simulink model "SAME5xPIM_MCLV2_MotorControl_ExtMode"  (R2021a)
settings: Solver=FixedStepDiscrete  StartTime=0.0  StopTime=inf  FixedStep=5e-5  RelTol=1e-3  EnableMultiTasking=on
InitFcn:
  | % DC Voltage
  | VDC = 24;
  | 
  | % Intersective PMW
  | Vmax = VDC/2;
  | Imax = 4;
  | 
  | Ts = 1e-4;
  | 
  | 
  | % pole paires
  | p = 4;
  | 
  | % QEI
  | lines = 4*1000;
  | eleclines = lines/p;
  | inveleclines = 1/eleclines
  | gainQEIspeed = 2*pi/Ts/lines
  | 
  | % Electrical parameters
  | R=0.656; L=0.35e-3; Phif=0.0066;
  | % Mechanical parameters
  | F=1.e-05; J=1e-05; C0 = 0.01;%10;%1;
undefined symbols (not defined in the file or in its folder): ADC0, AIN0, AIN6, B27, DiscIntNeverNeededParam, PA02, PA03, PA06, PA08, PA09, PA10, PA11, PA12, PA13, PA16, PA17, PA18, pad0, pad1, pad2, pad3, PB08, PC16, PC17, PC18, Pin, SAME54P20A, TQFP128, VREFA, wo0, wo1, wo2, wo4, wo5, wo6
libraries: simulink x15, MCHP_Blockset x9, dsparch4 x1
(part 2 of 2)

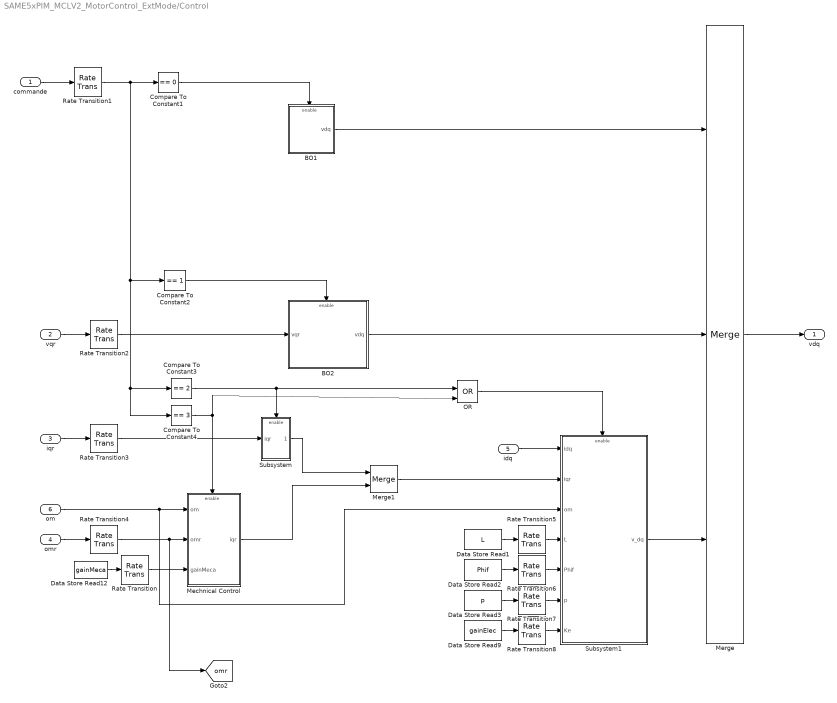
== system SAME5xPIM_MCLV2_MotorControl_ExtMode/Control ==
  commande : Inport
  vqr : Inport  Port=2
  iqr : Inport  Port=3
  omr : Inport  Port=4
  idq : Inport  Port=5
  om : Inport  Port=6
  BO1 : Subsystem
  BO2 : Subsystem
  Compare To Constant1 : simulink/Logic and Bit Operations/Compare To Constant  relop===  const=0  OutDataTypeStr=boolean
  Compare To Constant2 : simulink/Logic and Bit Operations/Compare To Constant  relop===  const=1  OutDataTypeStr=boolean
  Compare To Constant3 : simulink/Logic and Bit Operations/Compare To Constant  relop===  const=2  OutDataTypeStr=boolean
  Compare To Constant4 : simulink/Logic and Bit Operations/Compare To Constant  relop===  const=3  OutDataTypeStr=boolean
  Data Store Read1 : DataStoreRead  DataStoreName=L  SampleTime=1  IndexOptions=Index vector (dialog)  Indices=1  OutputSizes=1
  Data Store Read12 : DataStoreRead  DataStoreName=gainMeca  SampleTime=1  IndexOptions=Index vector (dialog)  Indices=1  OutputSizes=1
  Data Store Read2 : DataStoreRead  DataStoreName=Phif  SampleTime=1  IndexOptions=Index vector (dialog)  Indices=1  OutputSizes=1
  Data Store Read3 : DataStoreRead  DataStoreName=p  SampleTime=1  IndexOptions=Index vector (dialog)  Indices=1  OutputSizes=1
  Data Store Read9 : DataStoreRead  DataStoreName=gainElec  SampleTime=1  IndexOptions=Index vector (dialog)  Indices=1  OutputSizes=1
  Mechnical Control : Subsystem
  Merge : Merge  Inputs=3
  Merge1 : Merge
  OR : Logic  Operator=OR  IconShape=distinctive  AllPortsSameDT=off  OutDataTypeStr=boolean
  Rate Transition{,1..8} (9 alike) : RateTransition
  Subsystem : Subsystem
  Subsystem1 : Subsystem
  vdq : Outport  VectorParamsAs1DForOutWhenUnconnected=off
  tag scope: omr=global
  wires:
  Data Store Read12/1 -> Rate Transition/1
  omr/1 -> Rate Transition4/1
  iqr/1 -> Rate Transition3/1
  vqr/1 -> Rate Transition2/1
  Data Store Read2/1 -> Rate Transition6/1
  Data Store Read3/1 -> Rate Transition7/1
  Data Store Read1/1 -> Rate Transition5/1
  Data Store Read9/1 -> Rate Transition8/1
  BO2/1(vdq) -> Merge/2
  BO1/1(vdq) -> Merge/1
  Compare To Constant2/1 -> BO2/Enable
  Merge/1 -> vdq/1
  commande/1 -> Rate Transition1/1
  Compare To Constant1/1 -> BO1/Enable
  Compare To Constant3/1 -> OR/1, Subsystem/Enable
  Rate Transition1/1 -> Compare To Constant2/1, Compare To Constant3/1, Compare To Constant4/1, Compare To Constant1/1
  Subsystem/1(Out1) -> Merge1/1
  Mechnical Control/1(iqr) -> Merge1/2
  Compare To Constant4/1 -> OR/2, Mechnical Control/Enable
  om/1 -> Subsystem1/3(om), Mechnical Control/1(om)
  OR/1 -> Subsystem1/Enable
  idq/1 -> Subsystem1/1(idq)
  Merge1/1 -> Subsystem1/2(iqr)
  Subsystem1/1(v_dq) -> Merge/3
  Rate Transition2/1 -> BO2/1(vqr)
  Rate Transition3/1 -> Subsystem/1(iqr)
  Rate Transition4/1 -> Mechnical Control/2(omr), [omr]
  Rate Transition/1 -> Mechnical Control/3(gainMeca)
  Rate Transition5/1 -> Subsystem1/4(L)
  Rate Transition6/1 -> Subsystem1/5(Phif)
  Rate Transition7/1 -> Subsystem1/6(p)
  Rate Transition8/1 -> Subsystem1/7(Ke)

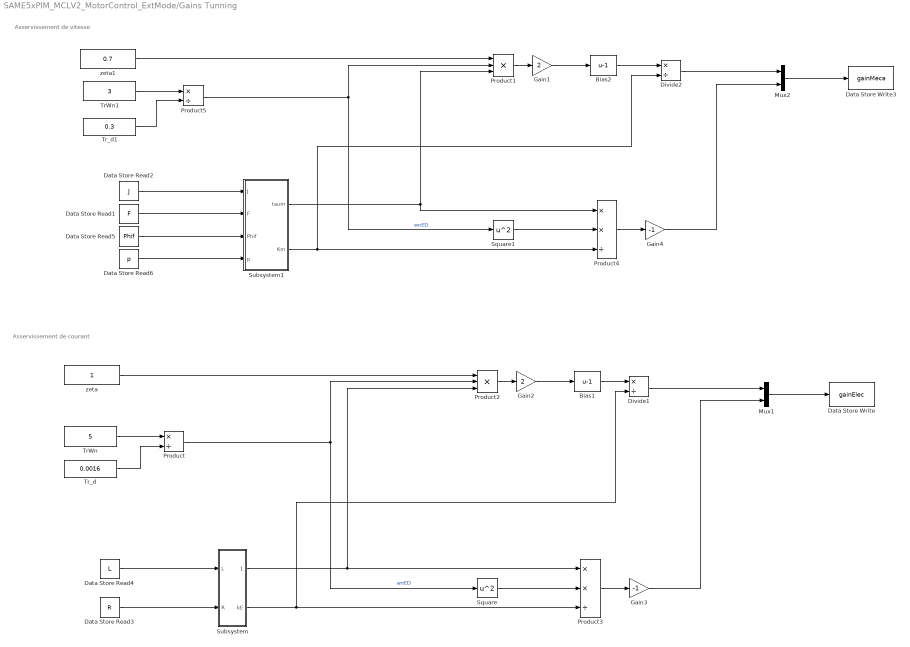
== system SAME5xPIM_MCLV2_MotorControl_ExtMode/Gains Tunning ==
  note: Asservissement de vitesse
  note: Asservissement de courant
  Bias1 : Bias  Bias=-1
  Bias2 : Bias  Bias=-1
  Data Store Read1 : DataStoreRead  DataStoreName=F  SampleTime=1  IndexOptions=Index vector (dialog)  Indices=1  OutputSizes=1
  Data Store Read2 : DataStoreRead  DataStoreName=J  SampleTime=1  IndexOptions=Index vector (dialog)  Indices=1  OutputSizes=1
  Data Store Read3 : DataStoreRead  DataStoreName=R  SampleTime=1  IndexOptions=Index vector (dialog)  Indices=1  OutputSizes=1
  Data Store Read4 : DataStoreRead  DataStoreName=L  SampleTime=1  IndexOptions=Index vector (dialog)  Indices=1  OutputSizes=1
  Data Store Read5 : DataStoreRead  DataStoreName=Phif  SampleTime=1  IndexOptions=Index vector (dialog)  Indices=1  OutputSizes=1
  Data Store Read6 : DataStoreRead  DataStoreName=p  SampleTime=1  IndexOptions=Index vector (dialog)  Indices=1  OutputSizes=1
  Data Store Write : DataStoreWrite  DataStoreName=gainElec  SampleTime=1  IndexOptions=Index vector (dialog)  Indices=1  OutputSizes=1
  Data Store Write3 : DataStoreWrite  DataStoreName=gainMeca  IndexOptions=Index vector (dialog)  Indices=1  OutputSizes=1
  Divide1 : Product  Inputs=*/
  Divide2 : Product  Inputs=*/
  Gain1 : Gain  Gain=2
  Gain2 : Gain  Gain=2
  Gain3 : Gain  Gain=-1
  Gain4 : Gain  Gain=-1
  Mux1 : Mux  Inputs=2
  Mux2 : Mux  Inputs=2
  Product : Product  Inputs=*/
  Product1 : Product  Inputs=3
  Product2 : Product  Inputs=3
  Product3 : Product  Inputs=**/
  Product4 : Product  Inputs=**/
  Product5 : Product  Inputs=*/
  Square : Math  Operator=square  SaturateOnIntegerOverflow=on
  Square1 : Math  Operator=square  SaturateOnIntegerOverflow=on
  Subsystem : Subsystem
  Subsystem1 : Subsystem
  TrWn : Constant  Value=5  OutDataTypeStr=single
  TrWn1 : Constant  Value=3  OutDataTypeStr=single
  Tr_d : Constant  Value=0.0016  OutDataTypeStr=single
  Tr_d1 : Constant  Value=0.3  OutDataTypeStr=single
  zeta : Constant  OutDataTypeStr=single
  zeta1 : Constant  Value=0.7  OutDataTypeStr=single
  wires:
  Subsystem1/2(Km) -> Product4/3, Divide2/2
  Subsystem1/1(taum) -> Product1/3, Product4/1
  Product5/1 -> Product1/2, Square1/1  "wnED"
  zeta1/1 -> Product1/1
  TrWn1/1 -> Product5/1
  Tr_d1/1 -> Product5/2
  Data Store Read6/1 -> Subsystem1/4(p)
  Data Store Read5/1 -> Subsystem1/3(Phif)
  Data Store Read1/1 -> Subsystem1/2(F)
  Data Store Read2/1 -> Subsystem1/1(J)
  Mux2/1 -> Data Store Write3/1
  Gain4/1 -> Mux2/2
  Product4/1 -> Gain4/1
  Divide2/1 -> Mux2/1
  Bias2/1 -> Divide2/1
  Product1/1 -> Gain1/1
  Gain1/1 -> Bias2/1
  Square1/1 -> Product4/2
  Square/1 -> Product3/2
  zeta/1 -> Product2/1
  Gain2/1 -> Bias1/1
  Subsystem/2(kE) -> Product3/3, Divide1/2
  Product/1 -> Square/1, Product2/2  "wnED"
  Tr_d/1 -> Product/2
  TrWn/1 -> Product/1
  Subsystem/1(tauE) -> Product3/1, Product2/3
  Data Store Read3/1 -> Subsystem/2(R)
  Data Store Read4/1 -> Subsystem/1(L)
  Mux1/1 -> Data Store Write/1
  Product2/1 -> Gain2/1
  Bias1/1 -> Divide1/1
  Divide1/1 -> Mux1/1
  Product3/1 -> Gain3/1
  Gain3/1 -> Mux1/2

== system SAME5xPIM_MCLV2_MotorControl_ExtMode/Inv Park ==
  cossin : Inport
  vdq : Inport  Port=2  PortDimensions=2
  Clakeinv : Subsystem
  ParkInv : Subsystem
  vabc : Outport  VectorParamsAs1DForOutWhenUnconnected=off
  wires:
  Clakeinv/1(abc) -> vabc/1
  ParkInv/1(valbe) -> Clakeinv/1(alphabeta)
  cossin/1 -> ParkInv/1(cos(pth)sin(pth))
  vdq/1 -> ParkInv/2(vdq)

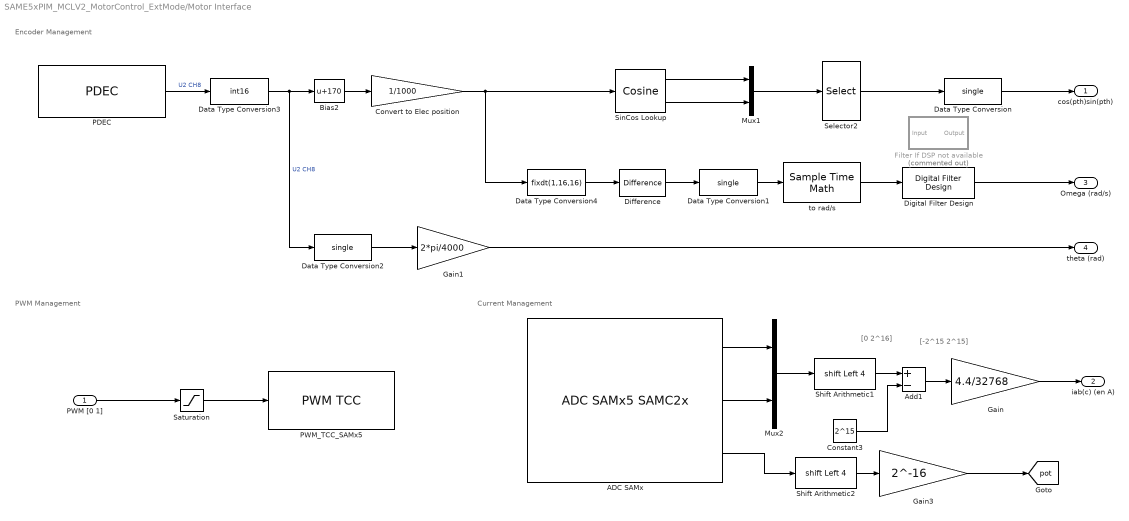
== system SAME5xPIM_MCLV2_MotorControl_ExtMode/Motor Interface ==
  note: Current Management
  note: [-2^15 2^15]
  note: [0 2^16]
  note: PWM Management
  note: Encoder Management
  PWM [0 1] : Inport
  ADC SAMx : MCHP_Blockset/Analog IO/ADC SAMx5 SAMC2x  ADCREF=ADC 0 and ADC 1 (slave)  VREF_seq0=Dynamic Options  VREF_seq0_TXT=PA03 / VREFA / Pin[10]  info=0  SampleTime=1e-4  MCHP_PORT={ADC0_seq0.0}{ADC0_AIN0}15:2:P2;{ADC0_seq1.0}{ADC0_AIN6}15:2:P6;{ADC1_seq0.0}{ADC1_AIN0}15:2:P40;  MCHP_MASTERLINK=SAME5xPIM_MCLV2_MotorControl_ExtMode/Microchip Master  MCHP_CRC=4644056  TrigSource_seq0=Dynamic Options  TrigSource_seq0_TXT=TCC0 PWM event Overflow - Period  ADC0_seq0=Dynamic Options  ADC0_seq0_TXT=PA02 / AIN0 / Pin[9]  ADC1_seq0=Dynamic Options  ADC1_seq0_TXT=PB08 / AIN0 / Pin[19]  ADC0_seq0_1=Dynamic Options  ADC0_seq0_1_TXT=Not Used  ADC1_seq0_1=Dynamic Options  ADC1_seq0_1_TXT=Not Used  ADC0_seq0_2=Dynamic Options  ADC0_seq0_2_TXT=Not Used  ADC1_seq0_2=Dynamic Options  ADC1_seq0_2_TXT=Not Used  ADC0_seq0_3=Dynamic Options  ADC0_seq0_3_TXT=Not Used  ADC1_seq0_3=Dynamic Options  ADC1_seq0_3_TXT=Not Used  ADC0_seq0_4=Dynamic Options  ADC0_seq0_4_TXT=Not Used  ADC1_seq0_4=Dynamic Options  ADC1_seq0_4_TXT=Not Used  ADC0_seq0_5=Dynamic Options  ADC0_seq0_5_TXT=Not Used  ADC1_seq0_5=Dynamic Options  ADC1_seq0_5_TXT=Not Used  Resolution_seq0=12 bits  SampleTime_seq0_s=1e-6  TrigTimeStep_seq0=on  info_seq0=0  TrigSource_seq1=Dynamic Options  TrigSource_seq1_TXT=after previous sequence  ADC0_seq1=Dynamic Options  ADC0_seq1_TXT=PA06 / AIN6 / Pin[23]  ADC1_seq1=Dynamic Options  ADC1_seq1_TXT=Not Used  ADC0_seq1_1=Dynamic Options  ADC0_seq1_1_TXT=Not Used  ADC1_seq1_1=Dynamic Options  ADC1_seq1_1_TXT=Not Used  ADC0_seq1_2=Dynamic Options  ADC0_seq1_2_TXT=Not Used  ADC1_seq1_2=Dynamic Options  ADC1_seq1_2_TXT=Not Used  ADC0_seq1_3=Dynamic Options  ADC0_seq1_3_TXT=Not Used  ADC1_seq1_3=Dynamic Options  ADC1_seq1_3_TXT=Not Used  ADC0_seq1_4=Dynamic Options  ADC0_seq1_4_TXT=Not Used  ADC1_seq1_4=Dynamic Options  ADC1_seq1_4_TXT=Not Used  ADC0_seq1_5=Dynamic Options  ADC0_seq1_5_TXT=Not Used  ADC1_seq1_5=Dynamic Options  ADC1_seq1_5_TXT=Not Used  Resolution_seq1=12 bits  SampleTime_seq1_s=1e-6  TrigTimeStep_seq1=off  info_seq1=0  TrigSource_seq2=Dynamic Options  TrigSource_seq2_TXT=after previous sequence  ADC0_seq2=Dynamic Options  ADC0_seq2_TXT=Not Used  ADC1_seq2=Dynamic Options  ADC1_seq2_TXT=Not Used  ADC0_seq2_1=Dynamic Options  ADC0_seq2_1_TXT=Not Used  ADC1_seq2_1=Dynamic Options  ADC1_seq2_1_TXT=Not Used  ADC0_seq2_2=Dynamic Options  ADC0_seq2_2_TXT=Not Used  ADC1_seq2_2=Dynamic Options  ADC1_seq2_2_TXT=Not Used  ADC0_seq2_3=Dynamic Options  ADC0_seq2_3_TXT=Not Used  ADC1_seq2_3=Dynamic Options  ADC1_seq2_3_TXT=Not Used  ADC0_seq2_4=Dynamic Options  ADC0_seq2_4_TXT=Not Used  ADC1_seq2_4=Dynamic Options  ADC1_seq2_4_TXT=Not Used  ADC0_seq2_5=Dynamic Options  ADC0_seq2_5_TXT=Not Used  ADC1_seq2_5=Dynamic Options  ADC1_seq2_5_TXT=Not Used  Resolution_seq2=12 bits  SampleTime_seq2_s=1e-6  TrigTimeStep_seq2=off  info_seq2=0  TrigSource_seq3=Dynamic Options  TrigSource_seq3_TXT=after previous sequence  ADC0_seq3=Dynamic Options  ADC0_seq3_TXT=Not Used  ADC1_seq3=Dynamic Options  ADC1_seq3_TXT=Not Used  ADC0_seq3_1=Dynamic Options  ADC0_seq3_1_TXT=Not Used  ADC1_seq3_1=Dynamic Options  ADC1_seq3_1_TXT=Not Used  ADC0_seq3_2=Dynamic Options  ADC0_seq3_2_TXT=Not Used  ADC1_seq3_2=Dynamic Options  ADC1_seq3_2_TXT=Not Used  ADC0_seq3_3=Dynamic Options  ADC0_seq3_3_TXT=Not Used  ADC1_seq3_3=Dynamic Options  ADC1_seq3_3_TXT=Not Used  ADC0_seq3_4=Dynamic Options  ADC0_seq3_4_TXT=Not Used  ADC1_seq3_4=Dynamic Options  ADC1_seq3_4_TXT=Not Used  ADC0_seq3_5=Dynamic Options  ADC0_seq3_5_TXT=Not Used  ADC1_seq3_5=Dynamic Options  ADC1_seq3_5_TXT=Not Used  Resolution_seq3=12 bits  SampleTime_seq3_s=1e-6  TrigTimeStep_seq3=off  info_seq3=0  TrigSource_seq4=Dynamic Options  TrigSource_seq4_TXT=after previous sequence  ADC0_seq4=Dynamic Options  ADC0_seq4_TXT=Not Used  ADC1_seq4=Dynamic Options  ADC1_seq4_TXT=Not Used  ADC0_seq4_1=Dynamic Options  ADC0_seq4_1_TXT=Not Used  ADC1_seq4_1=Dynamic Options  ADC1_seq4_1_TXT=Not Used  ADC0_seq4_2=Dynamic Options  ADC0_seq4_2_TXT=Not Used  ADC1_seq4_2=Dynamic Options  ADC1_seq4_2_TXT=Not Used  ADC0_seq4_3=Dynamic Options  ADC0_seq4_3_TXT=Not Used  ADC1_seq4_3=Dynamic Options  ADC1_seq4_3_TXT=Not Used  ADC0_seq4_4=Dynamic Options  ADC0_seq4_4_TXT=Not Used  ADC1_seq4_4=Dynamic Options  ADC1_seq4_4_TXT=Not Used  ADC0_seq4_5=Dynamic Options  ADC0_seq4_5_TXT=Not Used  ADC1_seq4_5=Dynamic Options  ADC1_seq4_5_TXT=Not Used  Resolution_seq4=12 bits  SampleTime_seq4_s=1e-6  TrigTimeStep_seq4=off  info_seq4=0  TrigSource_seq5=Dynamic Options  TrigSource_seq5_TXT=after previous sequence  ADC0_seq5=Dynamic Options  ADC0_seq5_TXT=Not Used  ADC1_seq5=Dynamic Options  ADC1_seq5_TXT=Not Used  ADC0_seq5_1=Dynamic Options  ADC0_seq5_1_TXT=Not Used  ADC1_seq5_1=Dynamic Options  ADC1_seq5_1_TXT=Not Used  ADC0_seq5_2=Dynamic Options  ADC0_seq5_2_TXT=Not Used  ADC1_seq5_2=Dynamic Options  ADC1_seq5_2_TXT=Not Used  ADC0_seq5_3=Dynamic Options  ADC0_seq5_3_TXT=Not Used  ADC1_seq5_3=Dynamic Options  ADC1_seq5_3_TXT=Not Used  ADC0_seq5_4=Dynamic Options  ADC0_seq5_4_TXT=Not Used  ADC1_seq5_4=Dynamic Options  ADC1_seq5_4_TXT=Not Used  ADC0_seq5_5=Dynamic Options  ADC0_seq5_5_TXT=Not Used  ADC1_seq5_5=Dynamic Options  ADC1_seq5_5_TXT=Not Used  Resolution_seq5=12 bits  SampleTime_seq5_s=1e-6  TrigTimeStep_seq5=off  info_seq5=0
      settings: SourceProductName=MPLAB Device Blocks for Simulink
  Add1 : Sum  Inputs=+-  OutDataTypeStr=single
  Bias2 : Bias  Bias=170
  Constant3 : Constant  Value=2^15  OutDataTypeStr=fixdt(0,16,0)
  Convert to Elec position : Gain  Gain=1/1000  OutDataTypeStr=fixdt(0,16,16)
  Data Type Conversion : DataTypeConversion  OutDataTypeStr=single
  Data Type Conversion1 : DataTypeConversion  OutDataTypeStr=single
  Data Type Conversion2 : DataTypeConversion  OutDataTypeStr=single
  Data Type Conversion3 : DataTypeConversion  OutDataTypeStr=int16  ConvertRealWorld=Stored Integer (SI)
  Data Type Conversion4 : DataTypeConversion  OutDataTypeStr=fixdt(1,16,16)  ConvertRealWorld=Stored Integer (SI)
  Difference : simulink/Discrete/Difference  ICPrevInput=0  OutMin=[]  OutMax=[]  OutDataType=fixdt(1, 16)  OutScaling=2^-10  DoSatur=off
  Digital Filter Design : dsparch4/Digital Filter Design  mwdsp_browser_bugfix_var=off
  Filter If DSP not available : Subsystem  Tag=FilterWizardSubSystem  Commented=on
      settings: ErrorFcn=dspFilterRealizedInBasicElemsAlgLoopErrFcnCallback
  Gain : Gain  Gain=4.4/32768
  Gain1 : Gain  Gain=2*pi/4000
  Gain3 : Gain  Gain=2^-16  OutDataTypeStr=single
  Mux1 : Mux  Inputs=2
  Mux2 : Mux  Inputs=2
  PDEC : MCHP_Blockset/QEI/PDEC  Mode=Quadrature Encoder  index=Reset counter  QDI0=PC16 / Pin[70]  QDI0_txt=Dynamic Options  QDI1=PC17 / Pin[71]  QDI1_txt=Dynamic Options  QDI2=PC18 / Pin[72]  QDI2_txt=Dynamic Options  maxCounterReset=-1  AutoCorrection=off  AutoCorrection_override=on  info=0  MCHP_MASTERLINK=SAME5xPIM_MCLV2_MotorControl_ExtMode/Microchip Master  SampleTime=1e-4  MCHP_PORT={PDEC A}{PDEC_QDI0}5:0:P80;{PDEC B}{PDEC_QDI1}5:0:P81;{PDEC index}{PDEC_QDI2}5:0:P82;  MAXPOS_INPUT=off  RESET_INPUT=off  OutputCounter=on  OutputCounter_Signed=unsigned  OutputRevolution=off  CounterRevolution_length=Counter is 13 bits ; revolution is 3 bits  OutputRevolution_Signed=unsigned  FILTER="250 (ns)  ->  freq 2 (MHz)"  FILTER_TXT="250 (ns)  ->  freq 2 (MHz)"  SWAP=off  QDI_invert_0=off  QDI_invert_1=off  QDI_invert_2=off
      settings: SourceProductName=MPLAB Device Blocks for Simulink
  PWM_TCC_SAMx5 : MCHP_Blockset/PWM IO/PWM TCC  TCCREF=TCC 0  WAVE_choice=Center aligned PWM  MaxPeriod_s=5e-5  OTMX=Default  WO0=Dynamic Options  WO0_TXT=PA08 / Pin[33] / wo0  WO1=Dynamic Options  WO1_TXT=PA09 / Pin[34] / wo1  WO2=Dynamic Options  WO2_TXT=PA10 / Pin[35] / wo2  WO3=Dynamic Options  WO3_TXT=Not Used  WO4=Dynamic Options  WO4_TXT=PA16 / Pin[66] / wo4  WO5=Dynamic Options  WO5_TXT=PA17 / Pin[67] / wo5  WO6=Dynamic Options  WO6_TXT=PA18 / Pin[68] / wo6  WO7=Dynamic Options  WO7_TXT=Not Used  info=0  evalin_ws=PWM0max=MCHP_Fun.Hex2num('40A76E0000000000');PWM0max=MCHP_Fun.Hex2num('40A76E0000000000');PWM0max=MCHP_Fun.Hex2num('40A76E0000000000');  SampleTime=1e-4  MCHP_PORT={PWM0_H0}{TCC0_WO0}5:1:P8;{PWM0_H1}{TCC0_WO1}5:1:P9;{PWM0_H2}{TCC0_WO2}5:1:P10;{PWM0_L0}{TCC0_WO4}5:1:P16;{PWM0_L1}{TCC0_WO5}5:1:P17;{PWM0_L2}{TCC0_WO6}5:1:P18;  MCHP_MASTERLINK=SAME5xPIM_MCLV2_MotorControl_ExtMode/Microchip Master  INVEN_WO0=off  INVEN_WO1=off  INVEN_WO2=off  INVEN_WO3=off  INVEN_WO4=off  INVEN_WO5=off  INVEN_WO6=off  INVEN_WO7=off  SWAP_PWM0=off  SWAP_PWM1=off  SWAP_PWM2=off  SWAP_PWM3=off  POL_PWM0=off  POL_PWM1=off  POL_PWM2=off  POL_PWM3=off  POL_PWM4=off  POL_PWM5=off  InitPeriod_s=5e-5  InitDutyCycle_s=2.5e-5  InitDeadTimeH_s=0.5e-6  InitDeadTimeL_s=0.5e-6  InitOutputOverride=0  InitOutputOverride_val=0  BlockInput_VectorScalar=Vectors (grouped by function)  BlockInput_Period=Not a block input  BlockInput_DutyCycle=a Floating Point input within range [0 1]  BlockInput_DeadTime=Not a block input  BlockInput_OutputOverride=Not a block input
      settings: SourceProductName=MPLAB Device Blocks for Simulink
  Saturation : Saturate  UpperLimit=0.98  LowerLimit=0.02  LinearizeAsGain=off  OutDataTypeStr=double
  Selector2 : Selector  InputPortWidth=2  IndexOptions=Index vector (dialog)  Indices=[2 1]  OutputSizes=1
  Shift Arithmetic1 : ArithShift  BitShiftNumber=4  BitShiftDirection=Left
  Shift Arithmetic2 : ArithShift  BitShiftNumber=4  BitShiftDirection=Left
  SinCos Lookup : simulink/Lookup Tables/Cosine  Formula=sin(2*pi*u) and cos(2*pi*u)  NumDataPoints=(2^12)+1  OutputWordLength=16  InternalRulePriority=Precision
      settings: SourceProductBaseCode=SL
  to rad/s : SampleTimeMath  TsampMathOp=/  weightValue=(4)/(2*pi)
  cos(pth)sin(pth) : Outport  VectorParamsAs1DForOutWhenUnconnected=off
  iab(c) (en A) : Outport  Port=2  VectorParamsAs1DForOutWhenUnconnected=off
  Omega (rad/s) : Outport  Port=3  PortDimensions=1  VectorParamsAs1DForOutWhenUnconnected=off
  theta (rad) : Outport  Port=4  VectorParamsAs1DForOutWhenUnconnected=off
  tag scope: pot=global
  wires:
  ADC SAMx/3 -> Shift Arithmetic2/1
  ADC SAMx/1 -> Mux2/1
  Constant3/1 -> Add1/2
  ADC SAMx/2 -> Mux2/2
  Shift Arithmetic1/1 -> Add1/1
  Mux2/1 -> Shift Arithmetic1/1
  Add1/1 -> Gain/1
  Gain3/1 -> [pot]
  Gain/1 -> iab(c) (en A)/1
  Shift Arithmetic2/1 -> Gain3/1
  Data Type Conversion1/1 -> to rad/s/1
  Data Type Conversion4/1 -> Difference/1
  Difference/1 -> Data Type Conversion1/1
  Gain1/1 -> theta (rad)/1
  Data Type Conversion2/1 -> Gain1/1
  Data Type Conversion3/1 -> Bias2/1, Data Type Conversion2/1  "U2 CH8"
  SinCos Lookup/1 -> Mux1/1
  SinCos Lookup/2 -> Mux1/2
  Selector2/1 -> Data Type Conversion/1
  Mux1/1 -> Selector2/1
  Data Type Conversion/1 -> cos(pth)sin(pth)/1
  Digital Filter Design/1 -> Omega (rad/s)/1
  PDEC/1 -> Data Type Conversion3/1  "U2 CH8"
  Bias2/1 -> Convert to Elec position/1
  to rad/s/1 -> Digital Filter Design/1
  Convert to Elec position/1 -> SinCos Lookup/1, Data Type Conversion4/1
  PWM [0 1]/1 -> Saturation/1
  Saturation/1 -> PWM_TCC_SAMx5/1

== system SAME5xPIM_MCLV2_MotorControl_ExtMode/PWM ==
  vabc : Inport
  50% average duty-cycle : Bias  Bias=0.5
  Gain : Gain  Gain=1/VDC  OutDataTypeStr=double
  PWM [0 1] : Outport  VectorParamsAs1DForOutWhenUnconnected=off
  wires:
  Gain/1 -> 50% average duty-cycle/1
  50% average duty-cycle/1 -> PWM [0 1]/1
  vabc/1 -> Gain/1

== system SAME5xPIM_MCLV2_MotorControl_ExtMode/Park  ==
  cossin : Inport
  xab(c) : Inport  Port=2
  Clark Fixe : Subsystem
  Park Fixe : Subsystem
  xdq : Outport  VectorParamsAs1DForOutWhenUnconnected=off
  wires:
  Park Fixe/1(xdq) -> xdq/1
  cossin/1 -> Park Fixe/2(cos(pth)sin(pth))
  xab(c)/1 -> Clark Fixe/1(xab(c))
  Clark Fixe/1(xalphabeta) -> Park Fixe/1(xalphabeta)

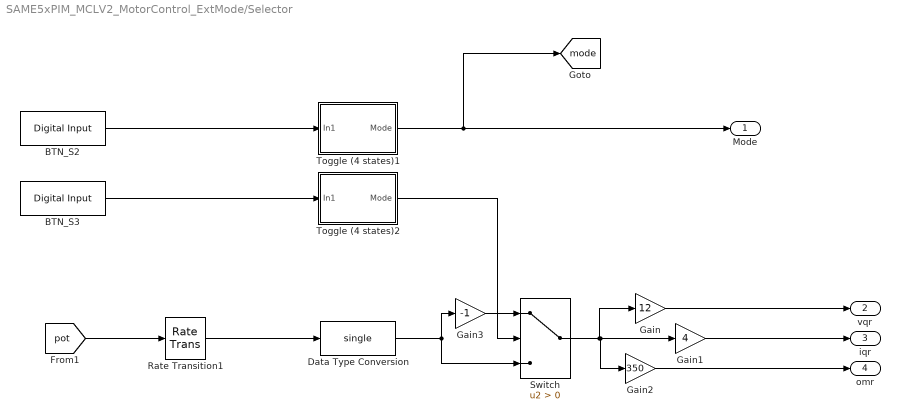
== system SAME5xPIM_MCLV2_MotorControl_ExtMode/Selector ==
  BTN_S2 : MCHP_Blockset/Digital IO/Digital Input  PORT=Dynamic Options  PORT_TXT="D   [ 0  1  8  9  10  11  12  20  21 ]"  PIN=9  PACK=off  SIMULTANEOUS=off  ORDERING=None  SampleTime=.1  MCHP_PORT={Digital In}{DIN}2:0:D9;  MCHP_MASTERLINK=SAME5xPIM_MCLV2_MotorControl_ExtMode/Microchip Master
      settings: SourceProductName=MPLAB Device Blocks for Simulink
  BTN_S3 : MCHP_Blockset/Digital IO/Digital Input  PORT=Dynamic Options  PORT_TXT="D   [ 0  1  8  9  10  11  12  20  21 ]"  PIN=10  PACK=off  SIMULTANEOUS=off  ORDERING=None  SampleTime=.1  MCHP_PORT={Digital In}{DIN}2:0:D10;  MCHP_MASTERLINK=SAME5xPIM_MCLV2_MotorControl_ExtMode/Microchip Master
      settings: SourceProductName=MPLAB Device Blocks for Simulink
  Data Type Conversion : DataTypeConversion  OutDataTypeStr=single
  Gain : Gain  Gain=12
  Gain1 : Gain  Gain=4
  Gain2 : Gain  Gain=350
  Gain3 : Gain  Gain=-1
  Rate Transition1 : RateTransition  OutPortSampleTime=0.1
  Switch : Switch  Criteria=u2 > Threshold
  Toggle (4 states)1 : Subsystem
  Toggle (4 states)2 : Subsystem
  Mode : Outport  VectorParamsAs1DForOutWhenUnconnected=off
  vqr : Outport  Port=2  VectorParamsAs1DForOutWhenUnconnected=off
  iqr : Outport  Port=3  VectorParamsAs1DForOutWhenUnconnected=off
  omr : Outport  Port=4  VectorParamsAs1DForOutWhenUnconnected=off
  tag scope: mode=global
  wires:
  Gain3/1 -> Switch/1
  Data Type Conversion/1 -> Switch/3, Gain3/1
  Toggle (4 states)2/1(Mode) -> Switch/2
  BTN_S3/1 -> Toggle (4 states)2/1(In1)
  Rate Transition1/1 -> Data Type Conversion/1
  [pot] -> Rate Transition1/1
  Toggle (4 states)1/1(Mode) -> Mode/1, [mode]
  Switch/1 -> Gain2/1, Gain1/1, Gain/1
  Gain/1 -> vqr/1
  Gain1/1 -> iqr/1
  Gain2/1 -> omr/1
  BTN_S2/1 -> Toggle (4 states)1/1(In1)

== system SAME5xPIM_MCLV2_MotorControl_ExtMode/Control/BO1 ==
  Enable : EnablePort
  Mux : Mux  Inputs=2
  vd : Constant  Value=0  OutMin=[-12]  OutMax=[12]  OutDataTypeStr=single
  vq : Constant  Value=0  OutMin=[-12]  OutMax=[12]  OutDataTypeStr=single
  vdq : Outport  VectorParamsAs1DForOutWhenUnconnected=off
  wires:
  vq/1 -> Mux/2
  Mux/1 -> vdq/1
  vd/1 -> Mux/1

== system SAME5xPIM_MCLV2_MotorControl_ExtMode/Control/BO2 ==
  vqr : Inport
  Enable : EnablePort
  Constant : Constant  Value=0  OutDataTypeStr=single
  Mux : Mux  Inputs=2
  vdq : Outport  VectorParamsAs1DForOutWhenUnconnected=off
  wires:
  Mux/1 -> vdq/1
  Constant/1 -> Mux/1
  vqr/1 -> Mux/2

== system SAME5xPIM_MCLV2_MotorControl_ExtMode/Control/Mechnical Control ==
  om : Inport
  omr : Inport  Port=2
  gainMeca : Inport  Port=3
  Enable : EnablePort  StatesWhenEnabling=reset
  Augmented state feedback : Subsystem
      settings: PortSchema="{\"entries\":[{\"content\":{\"sides\":[{\"content\":{\"connectorIds\":[\"In1\",\"In2\"]},\"type\":\"ConnectorPlacement.EquallySpacedRectSide\",\"uuid\":\"89137e2f-cd18-4dcc-a524-9caf5367be1f\"},{\"content\":{\"connectorIds\":[\"Out1\"],\"side\":\"RIGHT\"},\"type\":\"ConnectorPlacement.EquallySpacedRectSide\",\"uuid\":\"4fa0fb61-d5d6-47b2-9e74-7b8a54a26f7d\"},{\"content\":{\"connectorIds\":[],\"side\":\"TOP\"},\"type\":\"ConnectorPlacement.EquallySpacedRectSide\",\"uuid\":\"143a26d0-3cb3-43f1-872c-87316c90bc9f\"},{\"content\":{\"connectorIds\":[\"In3\"],\"side\":\"BOTTOM\"},\"type\":\"ConnectorPlacement.EquallySpacedRectSide\",\"uuid\":\"8516086b-4f00-45b1-b860-126256ccf69b\"},{\"content\":{\"connectorIds\":[],\"side\":\"HIDDEN\"},\"type\":\"ConnectorPlacement.EquallySpacedRectSide\",\"uuid\":\"abbfb321-16c4-4def-9c9f-eddb440e6971\"}]},\"type\":\"ConnectorPlacement.EquallySpacedConnector\",\"uuid\":\"ad3527e6-0bb9-4e51-b689-1365c7b23b5d\"}],\"packageUris\":[\"http://schema.mathworks.com/mf0/Connector/R2020b\"],\"version\":\"1.0\"}"
  iqr : Outport  VectorParamsAs1DForOutWhenUnconnected=off
  wires:
  gainMeca/1 -> Augmented state feedback/3(gainMeca)
  omr/1 -> Augmented state feedback/1(omref)
  Augmented state feedback/1(iqref) -> iqr/1
  om/1 -> Augmented state feedback/2(om)

== system SAME5xPIM_MCLV2_MotorControl_ExtMode/Control/Subsystem ==
  iqr : Inport
  Enable : EnablePort
  Out1 : Outport
  wires:
  iqr/1 -> Out1/1

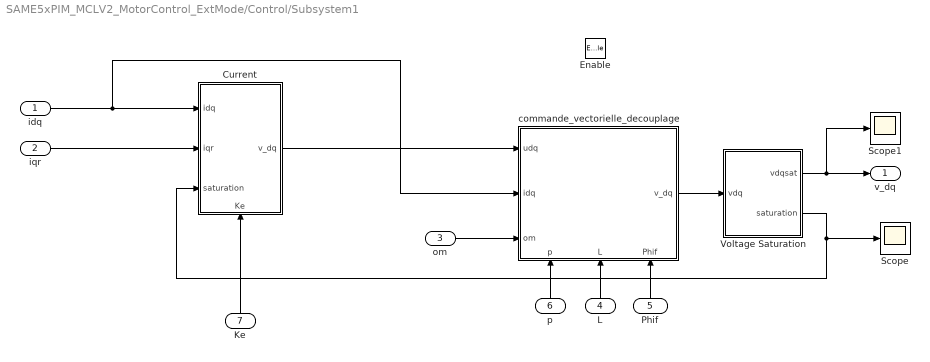
== system SAME5xPIM_MCLV2_MotorControl_ExtMode/Control/Subsystem1 ==
  idq : Inport
  iqr : Inport  Port=2
  om : Inport  Port=3
  L : Inport  Port=4
  Phif : Inport  Port=5
  p : Inport  Port=6
  Ke : Inport  Port=7
  Enable : EnablePort  StatesWhenEnabling=reset
  Current : Subsystem
      settings: PortSchema="{\"entries\":[{\"content\":{\"sides\":[{\"content\":{\"connectorIds\":[\"In1\",\"In2\",\"In3\"]},\"type\":\"ConnectorPlacement.EquallySpacedRectSide\",\"uuid\":\"0dd1bd5c-4f2d-4a51-9bc2-8bf74640d4ff\"},{\"content\":{\"connectorIds\":[\"Out1\"],\"side\":\"RIGHT\"},\"type\":\"ConnectorPlacement.EquallySpacedRectSide\",\"uuid\":\"9ff54608-efe8-47a2-97c0-1c2807ae0451\"},{\"content\":{\"connectorIds\":[],\"side\":\"TOP\"},\"type\":\"ConnectorPlacement.EquallySpacedRectSide\",\"uuid\":\"a5b0a1bc-2629-443b-a6ad-4c332df72e2c\"},{\"content\":{\"connectorIds\":[\"In4\"],\"side\":\"BOTTOM\"},\"type\":\"ConnectorPlacement.EquallySpacedRectSide\",\"uuid\":\"e8d63822-9705-4716-821c-9412f2966827\"},{\"content\":{\"connectorIds\":[],\"side\":\"HIDDEN\"},\"type\":\"ConnectorPlacement.EquallySpacedRectSide\",\"uuid\":\"63401b5c-75e9-49e9-aa08-12658d9987d3\"}]},\"type\":\"ConnectorPlacement.EquallySpacedConnector\",\"uuid\":\"d3f45542-3ea7-483a-a2ee-6c72d9ae8820\"}],\"packageUris\":[\"http://schema.mathworks.com/mf0/Connector/R2020b\"],\"version\":\"1.0\"}"
  Scope : Scope
  Scope1 : Scope
  Voltage Saturation : Subsystem
  commande_vectorielle_decouplage : Subsystem
      settings: PortSchema="{\"entries\":[{\"content\":{\"sides\":[{\"content\":{\"connectorIds\":[\"In1\",\"In2\",\"In3\"]},\"type\":\"ConnectorPlacement.EquallySpacedRectSide\",\"uuid\":\"169b5321-ee7c-423e-8449-192a786c9798\"},{\"content\":{\"connectorIds\":[\"Out1\"],\"side\":\"RIGHT\"},\"type\":\"ConnectorPlacement.EquallySpacedRectSide\",\"uuid\":\"910fdd05-0903-4759-8f85-a6669ffcf15d\"},{\"content\":{\"connectorIds\":[],\"side\":\"TOP\"},\"type\":\"ConnectorPlacement.EquallySpacedRectSide\",\"uuid\":\"8e0cf6ac-18cd-4e02-9312-1598b8dbe459\"},{\"content\":{\"connectorIds\":[\"In4\",\"In5\",\"In6\"],\"side\":\"BOTTOM\"},\"type\":\"ConnectorPlacement.EquallySpacedRectSide\",\"uuid\":\"bf7c0436-036d-4f64-97d8-e9b131650054\"},{\"content\":{\"connectorIds\":[],\"side\":\"HIDDEN\"},\"type\":\"ConnectorPlacement.EquallySpacedRectSide\",\"uuid\":\"cd87405f-25ee-425b-a181-6989070156fa\"}]},\"type\":\"ConnectorPlacement.EquallySpacedConnector\",\"uuid\":\"912b1b6f-c896-42c8-9325-248c15d73689\"}],\"packageUris\":[\"http://schema.mathworks.com/mf0/Connector/R2020b\"],\"version\":\"1.0\"}"
  v_dq : Outport
  wires:
  commande_vectorielle_decouplage/1(v_dq) -> Voltage Saturation/1(vdq)
  Voltage Saturation/2(saturation) -> Current/3(saturation), Scope/1
  Ke/1 -> Current/4(Ke)
  idq/1 -> Current/1(idq), commande_vectorielle_decouplage/2(idq)
  Current/1(v_dq) -> commande_vectorielle_decouplage/1(udq)
  iqr/1 -> Current/2(iqr)
  Voltage Saturation/1(vdqsat) -> v_dq/1, Scope1/1
  p/1 -> commande_vectorielle_decouplage/4(p)
  Phif/1 -> commande_vectorielle_decouplage/6(Phif)
  L/1 -> commande_vectorielle_decouplage/5(L)
  om/1 -> commande_vectorielle_decouplage/3(om)

== system SAME5xPIM_MCLV2_MotorControl_ExtMode/Gains Tunning/Subsystem ==
  L : Inport
  R : Inport  Port=2
  Divide1 : Product  Inputs=/
  Divide2 : Product  Inputs=*/
  tauE : Outport
  kE : Outport  Port=2
  wires:
  Divide1/1 -> kE/1  "kE"
  L/1 -> Divide2/1
  R/1 -> Divide2/2, Divide1/1
  Divide2/1 -> tauE/1  "tauE"

== system SAME5xPIM_MCLV2_MotorControl_ExtMode/Gains Tunning/Subsystem1 ==
  J : Inport
  F : Inport  Port=2
  Phif : Inport  Port=3
  p : Inport  Port=4
  Divide3 : Product  Inputs=*/
  Divide6 : Product  Inputs=*/
  Divide7 : Product  Inputs=**
  Gain : Gain  Gain=3/2
  taum : Outport
  Km : Outport  Port=2
  wires:
  Divide7/1 -> Divide3/1  "Km"
  Divide6/1 -> taum/1  "taum"
  Phif/1 -> Gain/1
  Divide3/1 -> Km/1  "Km"
  p/1 -> Divide7/2
  J/1 -> Divide6/1
  F/1 -> Divide6/2, Divide3/2
  Gain/1 -> Divide7/1

== system SAME5xPIM_MCLV2_MotorControl_ExtMode/Inv Park/Clakeinv ==
  alphabeta : Inport
  Clarke1 : Product  Multiplication=Matrix(*)  RndMeth=Simplest  OutDataTypeStr=Inherit: Same as first input
  Constant Magnitude : Constant  Value=[1 0 ; -1/2 sqrt(3)/2 ;-1/2 -sqrt(3)/2]'  OutDataTypeStr=Inherit: Inherit via back propagation  SampleTime=-1
  Math Function : Math  Operator=transpose  SignedPower=on  SaturateOnIntegerOverflow=on
  abc : Outport  VectorParamsAs1DForOutWhenUnconnected=off
  wires:
  Clarke1/1 -> abc/1
  Math Function/1 -> Clarke1/1
  Constant Magnitude/1 -> Clarke1/2
  alphabeta/1 -> Math Function/1

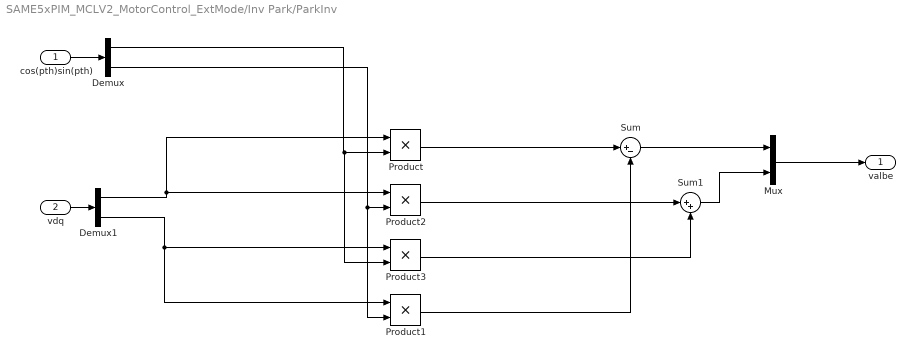
== system SAME5xPIM_MCLV2_MotorControl_ExtMode/Inv Park/ParkInv ==
  cos(pth)sin(pth) : Inport
  vdq : Inport  Port=2
  Demux : Demux  Outputs=2
  Demux1 : Demux  Outputs=2
  Mux : Mux  Inputs=2
  Product{,1..3} (4 alike) : Product
  Sum : Sum  Inputs=|+-
  Sum1 : Sum  Inputs=|++
  valbe : Outport  VectorParamsAs1DForOutWhenUnconnected=off
  wires:
  Product3/1 -> Sum1/2
  Product2/1 -> Sum1/1
  Mux/1 -> valbe/1
  Demux/2 -> Product1/2, Product2/2
  Demux/1 -> Product/2, Product3/2
  Product/1 -> Sum/1
  Product1/1 -> Sum/2
  Sum1/1 -> Mux/2
  Demux1/2 -> Product1/1, Product3/1
  Demux1/1 -> Product/1, Product2/1
  Sum/1 -> Mux/1
  cos(pth)sin(pth)/1 -> Demux/1
  vdq/1 -> Demux1/1

== system SAME5xPIM_MCLV2_MotorControl_ExtMode/Motor Interface/Filter If DSP not available ==
  Input : Inport
  Delay11 : Delay  DelayLength=1  InitialCondition=0
  Delay21 : Delay  DelayLength=1  InitialCondition=0
  SumA21 : Sum  Inputs=|+-  RndMeth=Nearest  SaturateOnIntegerOverflow=on  OutDataTypeStr=Inherit: Same as first input
  SumA31 : Sum  Inputs=|+-  RndMeth=Nearest  SaturateOnIntegerOverflow=on  OutDataTypeStr=Inherit: Same as first input
  SumB21 : Sum  Inputs=|++  RndMeth=Nearest  SaturateOnIntegerOverflow=on  OutDataTypeStr=Inherit: Same as first input
  SumB31 : Sum  Inputs=|++  RndMeth=Nearest  SaturateOnIntegerOverflow=on  OutDataTypeStr=Inherit: Same as first input
  a(2)(1) : Gain  Gain=-1.14298050253990113  ParamDataTypeStr=double  RndMeth=Nearest  SaturateOnIntegerOverflow=on  OutDataTypeStr=Inherit: Same as input
  a(3)(1) : Gain  Gain=0.412801598096188771  ParamDataTypeStr=double  RndMeth=Nearest  SaturateOnIntegerOverflow=on  OutDataTypeStr=Inherit: Same as input
  b(2)(1) : Gain  Gain=2  ParamDataTypeStr=double  RndMeth=Nearest  SaturateOnIntegerOverflow=on  OutDataTypeStr=Inherit: Same as input
  s(1) : Gain  Gain=0.0674552738890718956  ParamDataTypeStr=double  RndMeth=Nearest  SaturateOnIntegerOverflow=on  OutDataTypeStr=Inherit: Same as input
  Output : Outport
  wires:
  Input/1 -> s(1)/1
  s(1)/1 -> SumA21/1
  SumA21/1 -> SumA31/1
  SumA31/1 -> SumB21/1, Delay11/1
  SumB21/1 -> SumB31/1
  SumB31/1 -> Output/1
  a(2)(1)/1 -> SumA21/2
  Delay11/1 -> a(2)(1)/1, b(2)(1)/1, Delay21/1
  b(2)(1)/1 -> SumB21/2
  a(3)(1)/1 -> SumA31/2
  Delay21/1 -> a(3)(1)/1, SumB31/2

== system SAME5xPIM_MCLV2_MotorControl_ExtMode/Park /Clark Fixe ==
  note: k = 2/3 : invariant Magnitude
  note: Input is a vector of 3 elements, 3rd element is not beeing used
  xab(c) : Inport
  Clarke1 : Product  Multiplication=Matrix(*)  OutDataTypeStr=single  RndMeth=Convergent  SaturateOnIntegerOverflow=on
  Constant Magnitude : Constant  Value=[1 0 ; 1/sqrt(3) 2/sqrt(3) ];  OutDataTypeStr=single
  xalphabeta : Outport  VectorParamsAs1DForOutWhenUnconnected=off
  wires:
  xab(c)/1 -> Clarke1/2
  Constant Magnitude/1 -> Clarke1/1
  Clarke1/1 -> xalphabeta/1

== system SAME5xPIM_MCLV2_MotorControl_ExtMode/Park /Park Fixe ==
  xalphabeta : Inport
  cos(pth)sin(pth) : Inport  Port=2
  Demux : Demux  Outputs=2
  Demux1 : Demux  Outputs=2
  Mux : Mux  Inputs=2
  Product{,1..3} (4 alike) : Product
  Sum : Sum  Inputs=|++  SaturateOnIntegerOverflow=on
  Sum1 : Sum  Inputs=|-+  SaturateOnIntegerOverflow=on
  xdq : Outport  VectorParamsAs1DForOutWhenUnconnected=off
  wires:
  xalphabeta/1 -> Demux/1
  Mux/1 -> xdq/1
  Sum/1 -> Mux/1
  Demux/1 -> Product/1, Product1/1
  Demux/2 -> Product2/1, Product3/1
  Sum1/1 -> Mux/2
  Product3/1 -> Sum/2
  Product/1 -> Sum/1
  Demux1/1 -> Product/2, Product2/2
  Demux1/2 -> Product1/2, Product3/2
  Product1/1 -> Sum1/1
  Product2/1 -> Sum1/2
  cos(pth)sin(pth)/1 -> Demux1/1

== system SAME5xPIM_MCLV2_MotorControl_ExtMode/Selector/Toggle (4 states)1 ==
  In1 : Inport
  Bitwise Operator : simulink/Logic and Bit Operations/Bitwise Operator  logicop=AND  UseBitMask=on  BitMask=3  BitMaskRealWorld=Stored Integer
  Change when button is pressed : simulink/Logic and Bit Operations/Detect Decrease  vinit=0.0  OutDataTypeStr=uint8
  Sum : Sum  AccumDataTypeStr=uint16  OutDataTypeStr=uint16
  Unit Delay : UnitDelay  SampleTime=-1  HasFrameUpgradeWarning=on
  Mode : Outport  VectorParamsAs1DForOutWhenUnconnected=off
  wires:
  In1/1 -> Change when button is pressed/1
  Sum/1 -> Bitwise Operator/1
  Unit Delay/1 -> Sum/2
  Bitwise Operator/1 -> Unit Delay/1, Mode/1
  Change when button is pressed/1 -> Sum/1

== system SAME5xPIM_MCLV2_MotorControl_ExtMode/Selector/Toggle (4 states)2 ==
  In1 : Inport
  Bitwise Operator : simulink/Logic and Bit Operations/Bitwise Operator  logicop=AND  UseBitMask=on  BitMask=1  BitMaskRealWorld=Stored Integer
  Change when button is pressed : simulink/Logic and Bit Operations/Detect Decrease  vinit=0.0  OutDataTypeStr=uint8
  Sum : Sum  AccumDataTypeStr=uint16  OutDataTypeStr=uint16
  Unit Delay : UnitDelay  SampleTime=-1  HasFrameUpgradeWarning=on
  Mode : Outport  VectorParamsAs1DForOutWhenUnconnected=off
  wires:
  Change when button is pressed/1 -> Sum/1
  Bitwise Operator/1 -> Mode/1, Unit Delay/1
  Unit Delay/1 -> Sum/2
  Sum/1 -> Bitwise Operator/1
  In1/1 -> Change when button is pressed/1

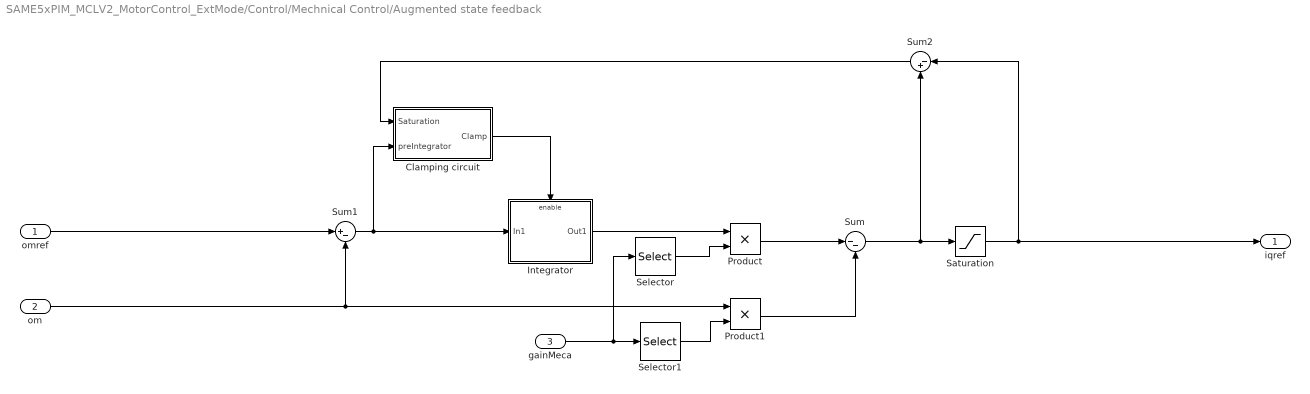
== system SAME5xPIM_MCLV2_MotorControl_ExtMode/Control/Mechnical Control/Augmented state feedback ==
  omref : Inport
  om : Inport  Port=2
  gainMeca : Inport  Port=3
  Clamping circuit : Subsystem
  Integrator : Subsystem
  Product : Product
  Product1 : Product
  Saturation : Saturate  UpperLimit=4  LowerLimit=-4
  Selector : Selector  InputPortWidth=2  IndexOptions=Index vector (dialog)  Indices=[2]  OutputSizes=1
  Selector1 : Selector  InputPortWidth=2  IndexOptions=Index vector (dialog)  Indices=1  OutputSizes=1
  Sum : Sum  Inputs=|--  OutDataTypeStr=single  SaturateOnIntegerOverflow=on
  Sum1 : Sum  Inputs=|+-
  Sum2 : Sum  Inputs=|-+  OutDataTypeStr=Inherit: Same as accumulator  SaturateOnIntegerOverflow=on
  iqref : Outport  VectorParamsAs1DForOutWhenUnconnected=off
  wires:
  gainMeca/1 -> Selector/1, Selector1/1
  Selector/1 -> Product/2
  Selector1/1 -> Product1/2
  Saturation/1 -> iqref/1, Sum2/1
  Integrator/1(Out1) -> Product/1
  Sum2/1 -> Clamping circuit/1(Saturation)
  Clamping circuit/1(Clamp) -> Integrator/Enable
  omref/1 -> Sum1/1
  Sum1/1 -> Clamping circuit/2(preIntegrator), Integrator/1(In1)
  om/1 -> Product1/1, Sum1/2
  Product/1 -> Sum/1
  Product1/1 -> Sum/2
  Sum/1 -> Saturation/1, Sum2/2

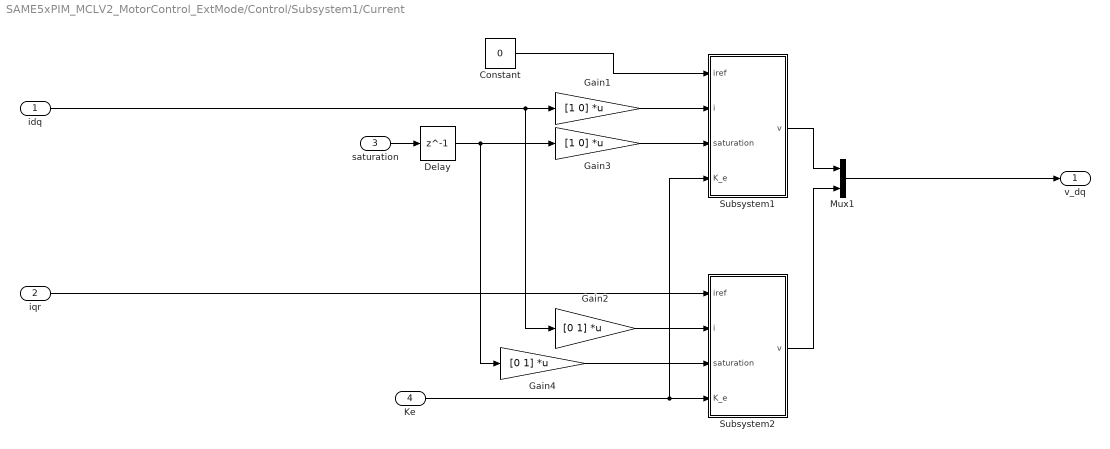
== system SAME5xPIM_MCLV2_MotorControl_ExtMode/Control/Subsystem1/Current ==
  idq : Inport
  iqr : Inport  Port=2
  saturation : Inport  Port=3
  Ke : Inport  Port=4
  Constant : Constant  Value=0
  Delay : Delay  DelayLength=1
  Gain1 : Gain  Gain=[1 0]  Multiplication=Matrix(K*u)  OutDataTypeStr=Inherit: Same as input
  Gain2 : Gain  Gain=[0 1]  Multiplication=Matrix(K*u)  OutDataTypeStr=Inherit: Same as input
  Gain3 : Gain  Gain=[1 0]  Multiplication=Matrix(K*u)  OutDataTypeStr=Inherit: Same as input
  Gain4 : Gain  Gain=[0 1]  Multiplication=Matrix(K*u)  OutDataTypeStr=Inherit: Same as input
  Mux1 : Mux  Inputs=2
  Subsystem1 : Subsystem
  Subsystem2 : Subsystem
  v_dq : Outport  VectorParamsAs1DForOutWhenUnconnected=off
  wires:
  iqr/1 -> Subsystem2/1(iref)
  Gain4/1 -> Subsystem2/3(saturation)
  Gain3/1 -> Subsystem1/3(saturation)
  Delay/1 -> Gain4/1, Gain3/1
  Ke/1 -> Subsystem2/4(K_e), Subsystem1/4(K_e)
  Mux1/1 -> v_dq/1
  Gain2/1 -> Subsystem2/2(i)
  Gain1/1 -> Subsystem1/2(i)
  idq/1 -> Gain1/1, Gain2/1
  Subsystem1/1(v) -> Mux1/1
  Subsystem2/1(v) -> Mux1/2
  saturation/1 -> Delay/1
  Constant/1 -> Subsystem1/1(iref)

== system SAME5xPIM_MCLV2_MotorControl_ExtMode/Control/Subsystem1/Voltage Saturation ==
  vdq : Inport
  Divide : Product  Inputs=*/
  Gain : Gain  Gain=Vmax
  Norm L2 : Subsystem
  Sum : Sum  Inputs=|+-
  Switch : Switch  Criteria=u2 > Threshold  Threshold=Vmax
  vdqsat : Outport  VectorParamsAs1DForOutWhenUnconnected=off
  saturation : Outport  Port=2  VectorParamsAs1DForOutWhenUnconnected=off
  wires:
  Gain/1 -> Switch/1
  Norm L2/1(y) -> Divide/2, Switch/2
  Divide/1 -> Gain/1
  Switch/1 -> Sum/2, vdqsat/1
  vdq/1 -> Norm L2/1(In1), Divide/1, Sum/1, Switch/3
  Sum/1 -> saturation/1

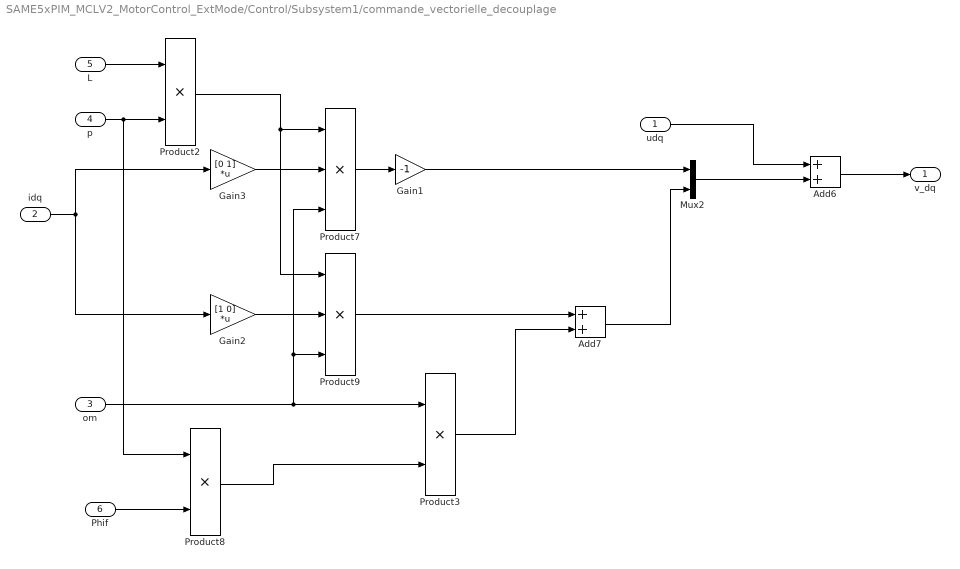
== system SAME5xPIM_MCLV2_MotorControl_ExtMode/Control/Subsystem1/commande_vectorielle_decouplage ==
  udq : Inport
  idq : Inport  Port=2
  om : Inport  Port=3
  p : Inport  Port=4
  L : Inport  Port=5
  Phif : Inport  Port=6
  Add6 : Sum
  Add7 : Sum
  Gain1 : Gain  Gain=-1
  Gain2 : Gain  Gain=[1 0]  Multiplication=Matrix(K*u)
  Gain3 : Gain  Gain=[0 1]  Multiplication=Matrix(K*u)
  Mux2 : Mux  Inputs=2
  Product2 : Product
  Product3 : Product
  Product7 : Product  Inputs=3
  Product8 : Product
  Product9 : Product  Inputs=3
  v_dq : Outport  VectorParamsAs1DForOutWhenUnconnected=off
  wires:
  Mux2/1 -> Add6/2
  Add7/1 -> Mux2/2
  udq/1 -> Add6/1
  Add6/1 -> v_dq/1
  idq/1 -> Gain2/1, Gain3/1
  Gain1/1 -> Mux2/1
  p/1 -> Product8/1, Product2/2
  L/1 -> Product2/1
  Product2/1 -> Product9/1, Product7/1
  Gain3/1 -> Product7/2
  Product7/1 -> Gain1/1
  Phif/1 -> Product8/2
  Product8/1 -> Product3/2
  om/1 -> Product3/1, Product9/3, Product7/3
  Gain2/1 -> Product9/2
  Product9/1 -> Add7/1
  Product3/1 -> Add7/2

== system SAME5xPIM_MCLV2_MotorControl_ExtMode/Control/Mechnical Control/Augmented state feedback/Clamping circuit ==
  note: The clamping enable or disable the integral action.
  Saturation : Inport  DisableCoverage=on
  preIntegrator : Inport  DisableCoverage=on  Port=2
  Compare To Zero1 : simulink/Logic and Bit Operations/Compare To Zero  relop=<=  OutDataTypeStr=boolean
  Delay : Delay  DelayLength=1  InitialCondition=0
  Multiply : Product
  Clamp : Outport  DisableCoverage=on  VectorParamsAs1DForOutWhenUnconnected=off
  wires:
  Compare To Zero1/1 -> Clamp/1
  preIntegrator/1 -> Multiply/2
  Multiply/1 -> Compare To Zero1/1
  Saturation/1 -> Delay/1
  Delay/1 -> Multiply/1

== system SAME5xPIM_MCLV2_MotorControl_ExtMode/Control/Mechnical Control/Augmented state feedback/Integrator ==
  In1 : Inport
  Enable : EnablePort
  Discrete-Time Integrator : DiscreteIntegrator  SampleTime=1e-4  OutDataTypeStr=single  SaturateOnIntegerOverflow=on  ICPrevOutput=DiscIntNeverNeededParam  ICPrevScaledInput=DiscIntNeverNeededParam
  Out1 : Outport  VectorParamsAs1DForOutWhenUnconnected=off
  wires:
  Discrete-Time Integrator/1 -> Out1/1
  In1/1 -> Discrete-Time Integrator/1

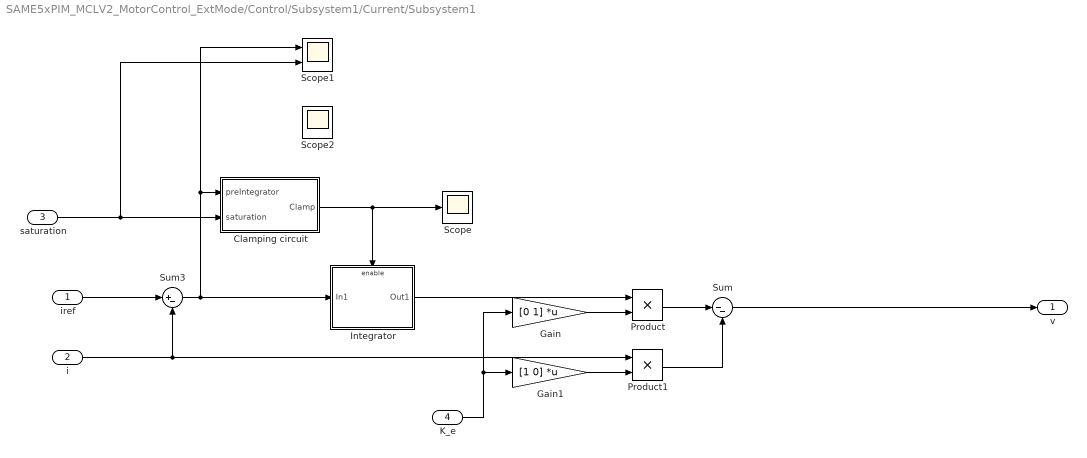
== system SAME5xPIM_MCLV2_MotorControl_ExtMode/Control/Subsystem1/Current/Subsystem1 ==
  iref : Inport
  i : Inport  Port=2
  saturation : Inport  Port=3
  K_e : Inport  Port=4
  Clamping circuit : Subsystem
  Gain : Gain  Gain=[0 1]  Multiplication=Matrix(K*u)
  Gain1 : Gain  Gain=[1 0]  Multiplication=Matrix(K*u)
  Integrator : Subsystem
  Product : Product
  Product1 : Product
  Scope : Scope
  Scope1 : Scope  NumInputPorts=2
  Scope2 : Scope
  Sum : Sum  Inputs=|--  OutDataTypeStr=single  SaturateOnIntegerOverflow=on
  Sum3 : Sum  Inputs=|+-
  v : Outport  VectorParamsAs1DForOutWhenUnconnected=off
  wires:
  saturation/1 -> Clamping circuit/2(saturation), Scope1/2
  Gain1/1 -> Product1/2
  Gain/1 -> Product/2
  K_e/1 -> Gain1/1, Gain/1
  Product1/1 -> Sum/2
  Product/1 -> Sum/1
  i/1 -> Product1/1, Sum3/2
  Sum3/1 -> Clamping circuit/1(preIntegrator), Scope1/1, Integrator/1(In1)
  iref/1 -> Sum3/1
  Clamping circuit/1(Clamp) -> Integrator/Enable, Scope/1
  Integrator/1(Out1) -> Product/1
  Sum/1 -> v/1

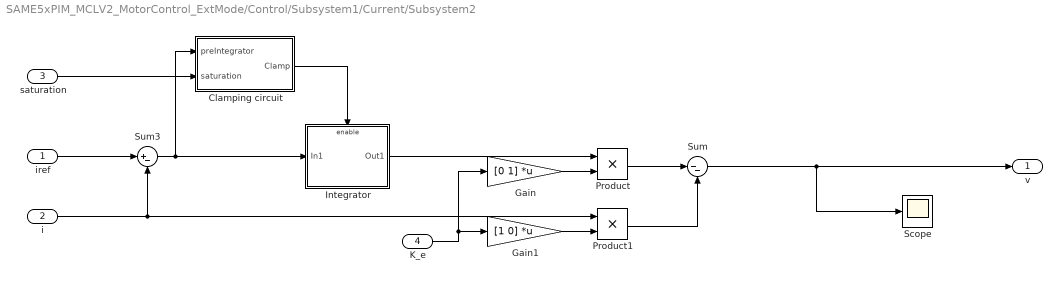
== system SAME5xPIM_MCLV2_MotorControl_ExtMode/Control/Subsystem1/Current/Subsystem2 ==
  iref : Inport
  i : Inport  Port=2
  saturation : Inport  Port=3
  K_e : Inport  Port=4
  Clamping circuit : Subsystem
  Gain : Gain  Gain=[0 1]  Multiplication=Matrix(K*u)
  Gain1 : Gain  Gain=[1 0]  Multiplication=Matrix(K*u)
  Integrator : Subsystem
  Product : Product
  Product1 : Product
  Scope : Scope
  Sum : Sum  Inputs=|--  OutDataTypeStr=single  SaturateOnIntegerOverflow=on
  Sum3 : Sum  Inputs=|+-
  v : Outport  VectorParamsAs1DForOutWhenUnconnected=off
  wires:
  Sum/1 -> v/1, Scope/1
  Integrator/1(Out1) -> Product/1
  Clamping circuit/1(Clamp) -> Integrator/Enable
  iref/1 -> Sum3/1
  Sum3/1 -> Integrator/1(In1), Clamping circuit/1(preIntegrator)
  i/1 -> Sum3/2, Product1/1
  Product/1 -> Sum/1
  Product1/1 -> Sum/2
  K_e/1 -> Gain/1, Gain1/1
  Gain/1 -> Product/2
  Gain1/1 -> Product1/2
  saturation/1 -> Clamping circuit/2(saturation)

== system SAME5xPIM_MCLV2_MotorControl_ExtMode/Control/Subsystem1/Voltage Saturation/Norm L2 ==
  In1 : Inport
  Dot Product : DotProduct  InputSameDT=on  OutDataTypeStr=Inherit: Inherit via internal rule
  Sqrt : Sqrt  SaturateOnIntegerOverflow=on
  y : Outport
  wires:
  Sqrt/1 -> y/1
  Dot Product/1 -> Sqrt/1
  In1/1 -> Dot Product/2, Dot Product/1

== system SAME5xPIM_MCLV2_MotorControl_ExtMode/Control/Subsystem1/Current/Subsystem1/Clamping circuit ==
  note: The clamping enable or disable the integral action.
  preIntegrator : Inport  DisableCoverage=on
  saturation : Inport  DisableCoverage=on  Port=2
  Compare To Zero1 : simulink/Logic and Bit Operations/Compare To Zero  relop=<=  OutDataTypeStr=boolean
  Multiply : Product
  Clamp : Outport  DisableCoverage=on  VectorParamsAs1DForOutWhenUnconnected=off
  wires:
  preIntegrator/1 -> Multiply/2
  Multiply/1 -> Compare To Zero1/1
  Compare To Zero1/1 -> Clamp/1
  saturation/1 -> Multiply/1

== system SAME5xPIM_MCLV2_MotorControl_ExtMode/Control/Subsystem1/Current/Subsystem1/Integrator ==
  In1 : Inport
  Enable : EnablePort
  Discrete-Time Integrator : DiscreteIntegrator  SampleTime=Ts  OutDataTypeStr=single  ICPrevOutput=DiscIntNeverNeededParam  ICPrevScaledInput=DiscIntNeverNeededParam
  Out1 : Outport  VectorParamsAs1DForOutWhenUnconnected=off
  wires:
  In1/1 -> Discrete-Time Integrator/1
  Discrete-Time Integrator/1 -> Out1/1

== system SAME5xPIM_MCLV2_MotorControl_ExtMode/Control/Subsystem1/Current/Subsystem2/Clamping circuit ==
  note: The clamping enable or disable the integral action.
  preIntegrator : Inport  DisableCoverage=on
  saturation : Inport  DisableCoverage=on  Port=2
  Compare To Zero1 : simulink/Logic and Bit Operations/Compare To Zero  relop=<=  OutDataTypeStr=boolean
  Multiply : Product
  Clamp : Outport  DisableCoverage=on  VectorParamsAs1DForOutWhenUnconnected=off
  wires:
  saturation/1 -> Multiply/1
  Compare To Zero1/1 -> Clamp/1
  Multiply/1 -> Compare To Zero1/1
  preIntegrator/1 -> Multiply/2

== system SAME5xPIM_MCLV2_MotorControl_ExtMode/Control/Subsystem1/Current/Subsystem2/Integrator ==
  In1 : Inport
  Enable : EnablePort
  Discrete-Time Integrator : DiscreteIntegrator  SampleTime=Ts  OutDataTypeStr=single  ICPrevOutput=DiscIntNeverNeededParam  ICPrevScaledInput=DiscIntNeverNeededParam
  Out1 : Outport  VectorParamsAs1DForOutWhenUnconnected=off
  wires:
  Discrete-Time Integrator/1 -> Out1/1
  In1/1 -> Discrete-Time Integrator/1
